simulink model "modelSS_temp"  (R2021b)
settings: Solver=VariableStepAuto  StartTime=0.0  StopTime=10000.0  RelTol=1e-3
undefined symbols (not defined in the file or in its folder): A, B, Bd, C, K, T_ambi_op
settings Model: Creator=martin  LastModifiedBy=kaspe

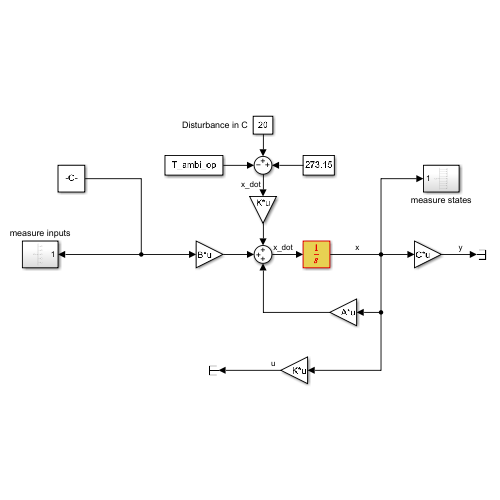
[thumbnail: Simulink's stored preview of the top-level diagram]
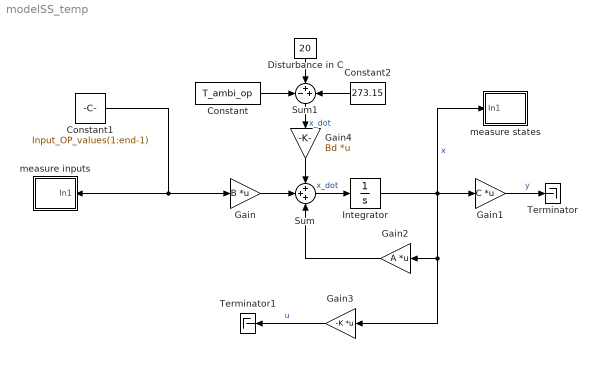
== system modelSS_temp ==
  Constant : Constant  Value=T_ambi_op
  Constant1 : Constant  Value=Input_OP_values(1:end-1)
  Constant2 : Constant  Value=273.15
  Disturbance in C : Constant  Value=20
  Gain : Gain  Gain=B  Multiplication=Matrix(K*u)
  Gain1 : Gain  Gain=C  Multiplication=Matrix(K*u)
  Gain2 : Gain  Gain=A  Multiplication=Matrix(K*u)
  Gain3 : Gain  Gain=-K  Multiplication=Matrix(K*u)
  Gain4 : Gain  Gain=Bd  Multiplication=Matrix(K*u)
  Integrator : Integrator  InitialCondition=ones(9,1)
  Sum : Sum  Inputs=+++
  Sum1 : Sum  Inputs=-++
  Terminator : Terminator
  Terminator1 : Terminator
  measure inputs : Subsystem
  measure states : Subsystem
  wires:
  Sum/1 -> Integrator/1  "x_dot"
  Integrator/1 -> measure states/1(In1), Gain3/1, Gain2/1, Gain1/1  "x"
  Gain2/1 -> Sum/3
  Gain/1 -> Sum/2
  Gain1/1 -> Terminator/1  "y"
  Gain4/1 -> Sum/1
  Sum1/1 -> Gain4/1  "x_dot"
  Constant/1 -> Sum1/1
  Disturbance in C/1 -> Sum1/2
  Constant2/1 -> Sum1/3
  Constant1/1 -> Gain/1, measure inputs/1(In1)
  Gain3/1 -> Terminator1/1  "u"

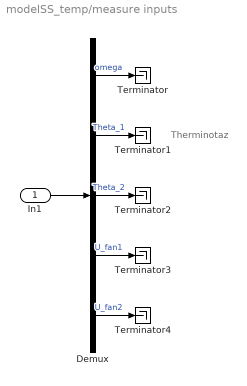
== system modelSS_temp/measure inputs ==
  note: Therminotaz
  In1 : Inport
  Demux : Demux  Outputs=5
  Terminator{,1..4} (5 alike) : Terminator
  wires:
  Demux/4 -> Terminator3/1  "U_fan1"
  Demux/2 -> Terminator1/1  "Theta_1"
  Demux/1 -> Terminator/1  "omega"
  Demux/3 -> Terminator2/1  "Theta_2"
  In1/1 -> Demux/1
  Demux/5 -> Terminator4/1  "U_fan2"

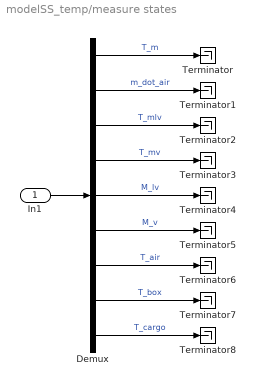
== system modelSS_temp/measure states ==
  In1 : Inport
  Demux : Demux  Outputs=9
  Terminator{,1..8} (9 alike) : Terminator
  wires:
  Demux/9 -> Terminator8/1  "T_cargo"
  Demux/8 -> Terminator7/1  "T_box"
  Demux/4 -> Terminator3/1  "T_mv"
  Demux/6 -> Terminator5/1  "M_v"
  Demux/1 -> Terminator/1  "T_m"
  Demux/7 -> Terminator6/1  "T_air"
  Demux/5 -> Terminator4/1  "M_lv"
  In1/1 -> Demux/1
  Demux/3 -> Terminator2/1  "T_mlv"
  Demux/2 -> Terminator1/1  "m_dot_air"
